simulink model "P_SP"  (R2022a)
settings: Solver=FixedStepAuto  StartTime=0.0  StopTime=25  FixedStep=0.001  RelTol=1e-3
libraries: cstblocks x2, simulink x2
settings Model: Creator=loryb  LastModifiedBy=loryb
settings SolverCC: ShapePreserveControl=EnableAll

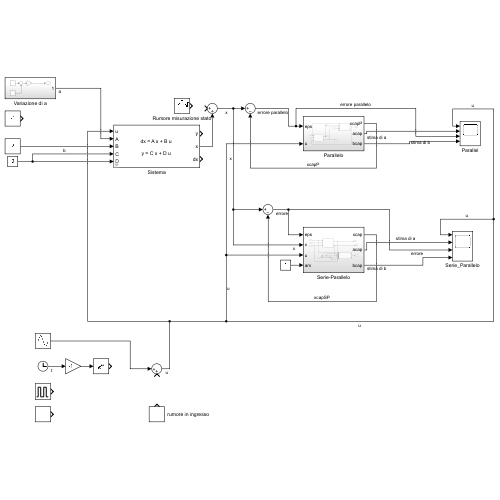
[thumbnail: Simulink's stored preview of the top-level diagram]
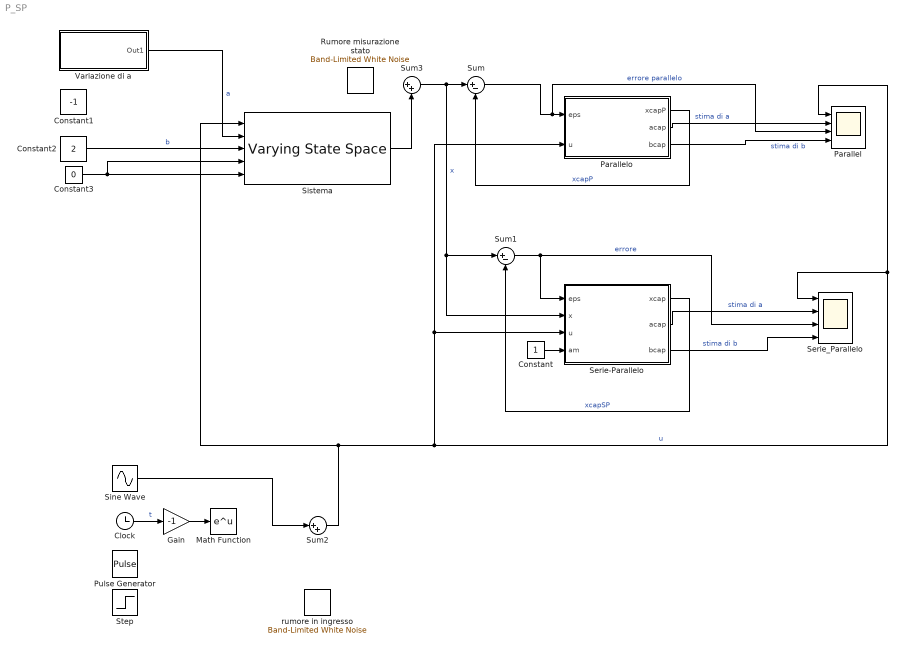
== system P_SP ==
  Clock : Clock
  Constant : Constant
  Constant1 : Constant  Value=-1
  Constant2 : Constant  Value=2
  Constant3 : Constant  Value=0
  Gain : Gain  Gain=-1
  Math Function : Math
  Parallel : Scope  NumInputPorts=4
  Parallelo : Subsystem
  Pulse Generator : DiscretePulseGenerator  PulseType=Time based  Period=5  PulseWidth=30
  Rumore misurazione stato : simulink/Sources/Band-Limited White Noise  Cov=[0.5]  Ts=0.1  seed=[23341]
  Serie-Parallelo : Subsystem
  Serie_Parallelo : Scope  NumInputPorts=4
  Sine Wave : Sin  SampleTime=0
  Sistema : cstblocks/Linear Parameter Varying/Varying State Space  x0=0  xNames=''  OutputX=on  OutputDX=on
  Step : Step  SampleTime=0
  Sum : Sum  Inputs=|+-
  Sum1 : Sum  Inputs=|+-
  Sum2 : Sum  Inputs=|++
  Sum3 : Sum  Inputs=|++
  Variazione di a : Subsystem
  rumore in ingresso : simulink/Sources/Band-Limited White Noise  Cov=[0.3]  Ts=0.1  seed=[23341]
  wires:
  Sistema/2 -> Sum3/2
  Constant2/1 -> Sistema/3  "b"
  Parallelo/1(xcapP) -> Sum/2  "xcapP"
  Parallelo/3(bcap) -> Parallel/4  "stima di b"
  Constant3/1 -> Sistema/4, Sistema/5
  Sum/1 -> Parallel/3, Parallelo/1(eps)  "errore parallelo"
  Constant/1 -> Serie-Parallelo/4(am)
  Serie-Parallelo/1(xcap) -> Sum1/2  "xcapSP"
  Serie-Parallelo/2(acap) -> Serie_Parallelo/2  "stima di a"
  Serie-Parallelo/3(bcap) -> Serie_Parallelo/4  "stima di b"
  Sum1/1 -> Serie_Parallelo/3, Serie-Parallelo/1(eps)  "errore"
  Sum2/1 -> Parallel/1, Serie_Parallelo/1, Serie-Parallelo/3(u), Parallelo/2(u), Sistema/1  "u"
  Gain/1 -> Math Function/1
  Clock/1 -> Gain/1  "t"
  Sum3/1 -> Serie-Parallelo/2(x), Sum1/1, Sum/1  "x"
  Parallelo/2(acap) -> Parallel/2  "stima di a"
  Sine Wave/1 -> Sum2/1
  Variazione di a/1(Out1) -> Sistema/2  "a"

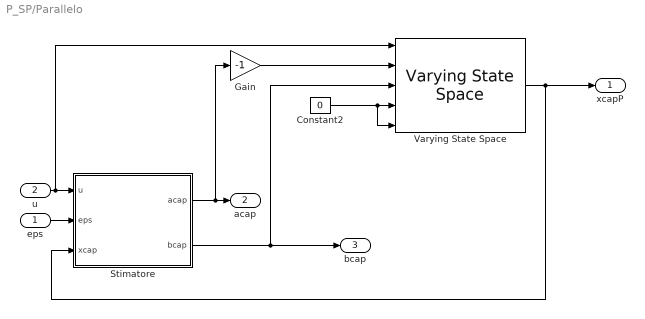
== system P_SP/Parallelo ==
  eps : Inport
  u : Inport  Port=2
  Constant2 : Constant  Value=0
  Gain : Gain  Gain=-1
  Stimatore : Subsystem
  Varying State Space : cstblocks/Linear Parameter Varying/Varying State Space  x0=0  xNames=''  OutputX=on  OutputDX=on
  xcapP : Outport
  acap : Outport  Port=2
  bcap : Outport  Port=3
  wires:
  Stimatore/2(bcap) -> Varying State Space/3, bcap/1
  u/1 -> Varying State Space/1, Stimatore/1(u)
  eps/1 -> Stimatore/2(eps)
  Stimatore/1(acap) -> Gain/1, acap/1
  Varying State Space/2 -> Stimatore/3(xcap), xcapP/1
  Constant2/1 -> Varying State Space/5, Varying State Space/4
  Gain/1 -> Varying State Space/2

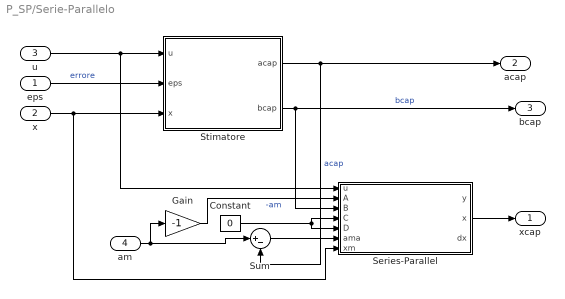
== system P_SP/Serie-Parallelo ==
  eps : Inport
  x : Inport  Port=2
  u : Inport  Port=3
  am : Inport  Port=4
  Constant : Constant  Value=0
  Gain : Gain  Gain=-1
  Series-Parallel : Subsystem  AncestorBlock=cstblocks/Linear Parameter Varying/Varying State Space  mask(Varying State Space){x0=0, xNames='', OutputX=on, OutputDX=on}
      mask prompts: x0 "Control:simulink:VaryingSSLabel1"; xNames "Control:simulink:VaryingSSLabel2"; OutputX "Control:simulink:VaryingSSLabel3"; OutputDX "Control:simulink:VaryingSSLabel4"
      mask help: Control:simulink:VaryingSS1
      mask init:
      | % Use exact linearization of product block
      | % pblks = find_system(gcb,'FollowLinks','on',...
      | %    'LookUnderMasks','all','SearchDepth',1,'BlockType','Product');
      | % rep = struct(...
      | %    'Specification','controllib.internal.blocks.matrixProductJacobian',...
      | %    'Type','Function',...
      | %    'ParameterNames','',...
      | %    'ParameterValues','');
      | % for i=1:numel(pblks)
      | %    set_param(pblks{i},...
      | %       'SCDEnableBlockLinearizationSpecification','on',...
      | %       'SCDBlockLinearizationSpecification',rep)
      | % end
      | SimStatus = get_param(bdroot,'SimulationStatus');
      | if any(strcmp(SimStatus,{'initializing','updating','stopped'}))
      |    varyingBlockMask('ss',gcb,OutputX,OutputDX)
      | end
      mask Help: eval('ctrlguihelp(''VaryingSSCT'');')
      mask DialogControl x0 Prompt: Initial conditions:
      mask DialogControl xNames Prompt: State names (e.g., 'position'):
      mask DialogControl OutputX Prompt: Output states
      mask DialogControl OutputDX Prompt: Output state derivatives
      mask Display:
      | port_label('input', 1, 'u')
      | port_label('input', 2, 'A')
      | port_label('input', 3, 'B')
      | port_label('input', 4, 'C')
      | port_label('input', 5, 'D')
      | port_label('output', 1, 'y')
      | next_ = 2;
      | if OutputX
      |    port_label('output', next_, 'x')
      |    next_ = next_+1;
      | end
      | if OutputDX
      |    port_label('output', next_, 'dx')
      |    next_ = next_+1;
      | end
      | text(0.5,0.65,'dx = A x + B u',...
      |    'horizontalAlignment', 'center','texmode','on')
      | text(0.5,0.35,'y = C x + D u',...
      |    'horizontalAlignment', 'center','texmode','on')
  Stimatore : Subsystem
  Sum : Sum  Inputs=|+-
  xcap : Outport
  acap : Outport  Port=2
  bcap : Outport  Port=3
  wires:
  x/1 -> Stimatore/3(x), Series-Parallel/7(xm)
  eps/1 -> Stimatore/2(eps)  "errore"
  u/1 -> Series-Parallel/1(u), Stimatore/1(u)
  Stimatore/2(bcap) -> bcap/1, Series-Parallel/3(B)  "bcap"
  Constant/1 -> Series-Parallel/4(C), Series-Parallel/5(D)
  Series-Parallel/2(x) -> xcap/1
  Stimatore/1(acap) -> Sum/2, acap/1  "acap"
  am/1 -> Gain/1, Sum/1
  Sum/1 -> Series-Parallel/6(ama)
  Gain/1 -> Series-Parallel/2(A)  "-am"

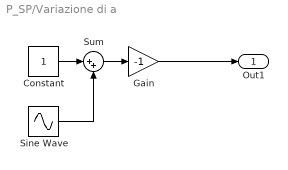
== system P_SP/Variazione di a ==
  Constant : Constant
  Gain : Gain  Gain=-1
  Sine Wave : Sin  Amplitude=0.1  Frequency=2*pi/(24*3600)  SampleTime=0
  Sum : Sum  Inputs=|++
  Out1 : Outport
  wires:
  Constant/1 -> Sum/1
  Sine Wave/1 -> Sum/2
  Gain/1 -> Out1/1
  Sum/1 -> Gain/1

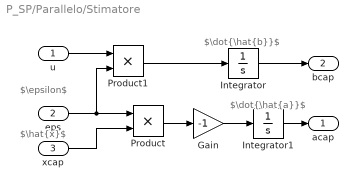
== system P_SP/Parallelo/Stimatore ==
  note: $\epsilon$
  note: $\dot{\hat{b}}$
  note: $\dot{\hat{a}}$
  note: $\hat{x}$
  u : Inport
  eps : Inport  Port=2
  xcap : Inport  Port=3
  Gain : Gain  Gain=-1
  Integrator : Integrator
  Integrator1 : Integrator
  Product : Product
  Product1 : Product
  acap : Outport
  bcap : Outport  Port=2
  wires:
  Product/1 -> Gain/1
  eps/1 -> Product1/2, Product/1
  xcap/1 -> Product/2
  u/1 -> Product1/1
  Product1/1 -> Integrator/1
  Integrator/1 -> bcap/1
  Gain/1 -> Integrator1/1
  Integrator1/1 -> acap/1

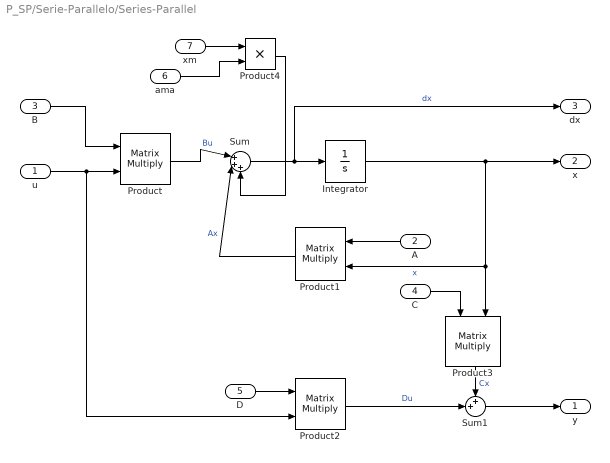
== system P_SP/Serie-Parallelo/Series-Parallel ==
  u : Inport
  A : Inport  Port=2
  B : Inport  Port=3
  C : Inport  Port=4
  D : Inport  Port=5
  ama : Inport  Port=6
  xm : Inport  Port=7
  Integrator : Integrator  InitialCondition=x0  ContinuousStateAttributes=xNames
  Product{,1..3} (4 alike) : Product  SCDEnableBlockLinearizationSpecification=on  Multiplication=Matrix(*)
  Product4 : Product
  Sum : Sum  Inputs=|+++
  Sum1 : Sum  Inputs=++|
  y : Outport  VectorParamsAs1DForOutWhenUnconnected=off
  x : Outport  Port=2  VectorParamsAs1DForOutWhenUnconnected=off
  dx : Outport  Port=3  VectorParamsAs1DForOutWhenUnconnected=off
  wires:
  C/1 -> Product3/1
  D/1 -> Product2/1
  u/1 -> Product2/2, Product/2
  A/1 -> Product1/1
  Product1/1 -> Sum/2  "Ax"
  B/1 -> Product/1
  Sum1/1 -> y/1
  Integrator/1 -> x/1, Product1/2, Product3/2  "x"
  Product2/1 -> Sum1/2  "Du"
  Product3/1 -> Sum1/1  "Cx"
  Sum/1 -> Integrator/1, dx/1  "dx"
  Product/1 -> Sum/1  "Bu"
  xm/1 -> Product4/1
  ama/1 -> Product4/2
  Product4/1 -> Sum/3

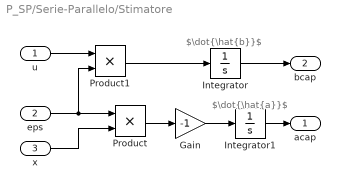
== system P_SP/Serie-Parallelo/Stimatore ==
  note: $\dot{\hat{b}}$
  note: $\dot{\hat{a}}$
  u : Inport
  eps : Inport  Port=2
  x : Inport  Port=3
  Gain : Gain  Gain=-1
  Integrator : Integrator
  Integrator1 : Integrator
  Product : Product
  Product1 : Product
  acap : Outport
  bcap : Outport  Port=2
  wires:
  Product/1 -> Gain/1
  eps/1 -> Product1/2, Product/1
  x/1 -> Product/2
  u/1 -> Product1/1
  Product1/1 -> Integrator/1
  Integrator/1 -> bcap/1
  Gain/1 -> Integrator1/1
  Integrator1/1 -> acap/1
